simulink model "Model"  (R2016a)
settings: Solver=ode3  StartTime=0.0  StopTime=inf  RelTol=1e-3
libraries: vexarmcortexlib x3
settings Model: ExtModeTrigDuration=25  Creator=Jonathan  LastModifiedBy=Windows7Ult
settings DataIOCC: LimitDataPoints=on  SignalLoggingSaveFormat=ModelDataLogs
settings OptimizationCC: ExpressionDepthLimit=2147483647  OptimizeModelRefInitCode=on  LifeSpan=Inf  MaxStackSize=64
settings DebuggingCC: UnderspecifiedInitializationDetection=Classic  MergeDetectMultiDrivingBlocksExec=none  InheritedTsInSrcMsg=none  FcnCallInpInsideContextMsg=UseLocalSettings  UnconnectedInputMsg=none  UnconnectedOutputMsg=none  StateNameClashWarn=warning
settings HardwareCC: ProdBitPerPointer=32  ProdLargestAtomicInteger=Long  ProdLargestAtomicFloat=Double  ProdIntDivRoundTo=Undefined  ProdWordSize=32  ProdHWDeviceType=ARM Compatible->ARM Cortex
settings ModelReferenceCC: PropagateSignalLabelsOutOfModel=off
settings RTWCC: SystemTargetFile=ert.tlc  HardwareBoard=ARM Cortex-based VEX Microcontroller  TemplateMakefile=ert_default_tmf  Toolchain=GNU Tools for VEX ARM Cortex
settings CodeAppCC: IgnoreCustomStorageClasses=off  CustomSymbolStrType=$N$R$M  InternalIdentifier=Classic
settings ERTTargetCC: CodeReplacementLibrary=GCC ARM Cortex-M3  ConvertIfToSwitch=off  SuppressUnreachableDefaultCases=off

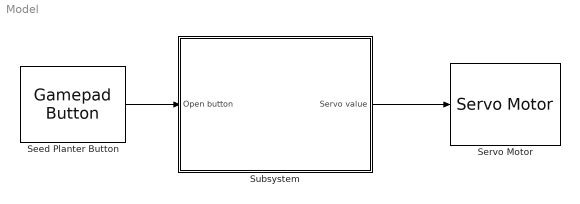
== system Model ==
  Seed Planter Button : vexarmcortexlib/Gamepad Button  joystick=1  chan=5  button56=Down  button78=Right  SimulationIn=off  sample_time=0.2
  Servo Motor : vexarmcortexlib/Servo Motor  motor=4  scaleFactor=90/127  SimulationOut=off
  Subsystem : Subsystem
  wires:
  Seed Planter Button/1 -> Subsystem/1(Open button)
  Subsystem/1(Servo value) -> Servo Motor/1

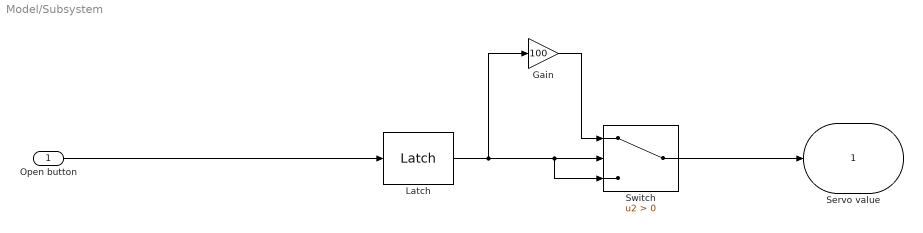
== system Model/Subsystem ==
  Open button : Inport
  Gain : Gain  Gain=100
  Latch : vexarmcortexlib/Utilities/Latch  output0=off
  Switch : Switch  Criteria=u2 > Threshold
  Servo value : Outport
  wires:
  Open button/1 -> Latch/1
  Latch/1 -> Gain/1, Switch/3, Switch/2
  Gain/1 -> Switch/1
  Switch/1 -> Servo value/1
